simulink model "simple_double_argon_mask"  (Simulink 7.7)
settings: Solver=ode15s  StartTime=0.0  StopTime=3600*24  RelTol=1e-3
libraries: fl_lib x38, nesl_utility x5
settings Model: Creator=jlanfrey  LastModifiedBy=Administrateur

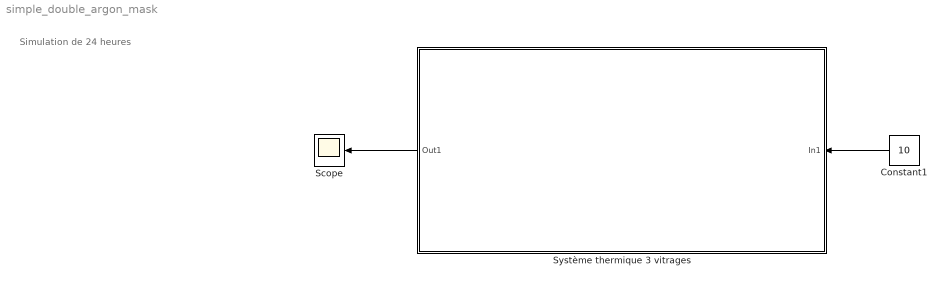
== system simple_double_argon_mask ==
  note: Simulation de 24 heures
  Constant1 : Constant  Value=10
  Scope : Scope
      settings: TimeRange=90000  YMin=14  YMax=20
  Système thermique 3 vitrages : Subsystem  mask{lf=0.6, hf=1, ev=4, ei=16, sp=10, hp=2.5, temp=20}
      mask prompts: lf "Largeur fenetre ? (m)"; hf "Hauteur fenetre ? (m)"; ev "Epaisseur d'un verre de la fenetre ? (mm)"; ei "Epaisseur isolant (air ou argon) ? (mm)"; sp "Suface pièce (m^2)"; hp "Hauteur pièce ? (m)"; temp "Température initiale (°C)"
      mask Display:
      | image(imread('vitrage.jpg'))
      | port_label('output', 1, 'Temp int')
      | port_label('input', 1, 'Temp exter')
  wires:
  Constant1/1 -> Système thermique 3 vitrages/1(In1)
  Système thermique 3 vitrages/1(Out1) -> Scope/1

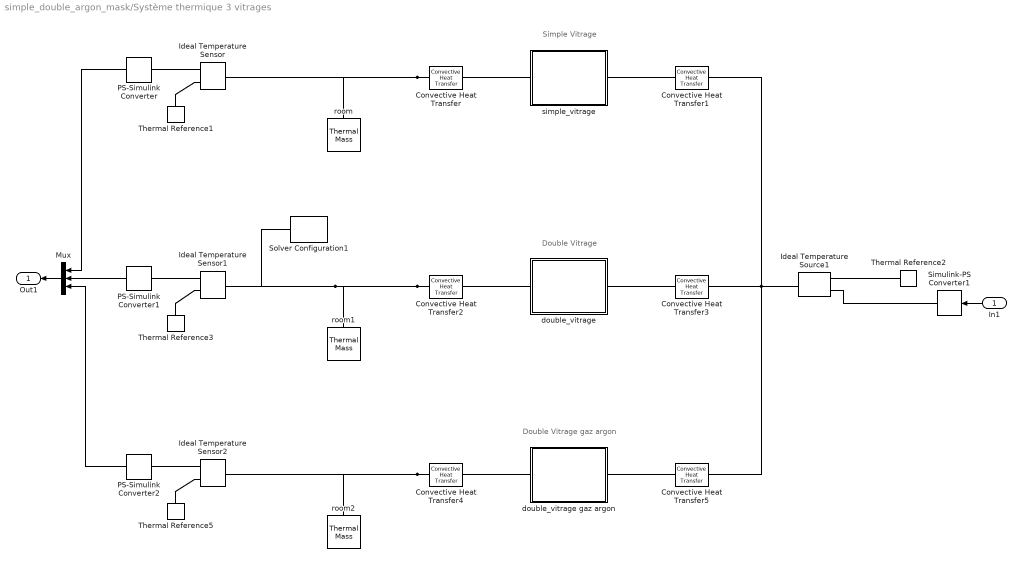
== system simple_double_argon_mask/Système thermique 3 vitrages ==
  note: Double Vitrage gaz argon
  note: Double Vitrage
  note: Simple Vitrage
  In1 : Inport
  Convective Heat Transfer : fl_lib/Thermal/Thermal Elements/Convective Heat Transfer  SystemSampleTime=-1  area=lf*hf m^2  heat_tr_coeff=1/0.13 W/(m^2 * K)  Q_Log=off  T_Log=off  LocalVarNames=|Q|T  LocalVarDescs=|Q|T  LocalVarLogging=[0 0]
  Convective Heat Transfer1 : fl_lib/Thermal/Thermal Elements/Convective Heat Transfer  SystemSampleTime=-1  area=lf*hf m^2  heat_tr_coeff=1/0.04 W/(m^2 * K)  Q_Log=off  T_Log=off  LocalVarNames=|Q|T  LocalVarDescs=|Q|T  LocalVarLogging=[0 0]
  Convective Heat Transfer2 : fl_lib/Thermal/Thermal Elements/Convective Heat Transfer  SystemSampleTime=-1  area=lf*hf m^2  heat_tr_coeff=1/0.13 W/(m^2 * K)  Q_Log=off  T_Log=off  LocalVarNames=|Q|T  LocalVarDescs=|Q|T  LocalVarLogging=[0 0]
  Convective Heat Transfer3 : fl_lib/Thermal/Thermal Elements/Convective Heat Transfer  SystemSampleTime=-1  area=lf*hf m^2  heat_tr_coeff=1/0.04 W/(m^2 * K)  Q_Log=off  T_Log=off  LocalVarNames=|Q|T  LocalVarDescs=|Q|T  LocalVarLogging=[0 0]
  Convective Heat Transfer4 : fl_lib/Thermal/Thermal Elements/Convective Heat Transfer  SystemSampleTime=-1  area=lf*hf m^2  heat_tr_coeff=1/0.13 W/(m^2 * K)  Q_Log=off  T_Log=off  LocalVarNames=|Q|T  LocalVarDescs=|Q|T  LocalVarLogging=[0 0]
  Convective Heat Transfer5 : fl_lib/Thermal/Thermal Elements/Convective Heat Transfer  SystemSampleTime=-1  area=lf*hf m^2  heat_tr_coeff=1/0.04 W/(m^2 * K)  Q_Log=off  T_Log=off  LocalVarNames=|Q|T  LocalVarDescs=|Q|T  LocalVarLogging=[0 0]
  Ideal Temperature Sensor : fl_lib/Thermal/Thermal Sensors/Ideal Temperature Sensor  SystemSampleTime=-1  Qs_Log=off  Ts_Log=off  LocalVarNames=|Qs|Ts  LocalVarDescs=|Qs|Ts  LocalVarLogging=[0 0]
  Ideal Temperature Sensor1 : fl_lib/Thermal/Thermal Sensors/Ideal Temperature Sensor  SystemSampleTime=-1  Qs_Log=off  Ts_Log=off  LocalVarNames=|Qs|Ts  LocalVarDescs=|Qs|Ts  LocalVarLogging=[0 0]
  Ideal Temperature Sensor2 : fl_lib/Thermal/Thermal Sensors/Ideal Temperature Sensor  SystemSampleTime=-1  Qs_Log=off  Ts_Log=off  LocalVarNames=|Qs|Ts  LocalVarDescs=|Qs|Ts  LocalVarLogging=[0 0]
  Ideal Temperature Source1 : fl_lib/Thermal/Thermal Sources/Ideal Temperature Source  SystemSampleTime=-1  Q_Log=off  T_Log=off  LocalVarNames=|Q|T  LocalVarDescs=|Q|T  LocalVarLogging=[0 0]
  Mux : Mux  Inputs=3
  PS-Simulink Converter : nesl_utility/PS-Simulink Converter  SystemSampleTime=-1  PhysicalDomain=network_engine_domain  LeftPortType=input  RightPortType=output  SubClassName=ps_output  Unit=C  AffineConversion=on
  PS-Simulink Converter1 : nesl_utility/PS-Simulink Converter  SystemSampleTime=-1  PhysicalDomain=network_engine_domain  LeftPortType=input  RightPortType=output  SubClassName=ps_output  Unit=C  AffineConversion=on
  PS-Simulink Converter2 : nesl_utility/PS-Simulink Converter  SystemSampleTime=-1  PhysicalDomain=network_engine_domain  LeftPortType=input  RightPortType=output  SubClassName=ps_output  Unit=C  AffineConversion=on
  Simulink-PS Converter1 : nesl_utility/Simulink-PS Converter  SystemSampleTime=-1  PhysicalDomain=network_engine_domain  LeftPortType=input  RightPortType=output  SubClassName=ps_input  Unit=C  AffineConversion=on  InputFilterTimeConstant=.001  UdotUserProvided=0
  Solver Configuration1 : nesl_utility/Solver Configuration  SystemSampleTime=-1  PhysicalDomain=network_engine_domain  LeftPortType=input  RightPortType=generic  SubClassName=solver  Accelerate=off  Profile=off  ResidualTolerance=1e-9  MaxNonlinIter=3  MaxModeIter=2  DoFixedCost=off  UseLocalSampling=off  DoDC=off  LinearAlgebra=Sparse  LocalSolverSampleTime=.001  LocalSolverChoice=NE_BACKWARD_EULER_ADVANCER  UseLocalSolver=off
  Thermal Reference{1..3,5} (4 alike) : fl_lib/Thermal/Thermal Elements/Thermal Reference  SystemSampleTime=-1  Q_Log=off  LocalVarNames=|Q  LocalVarDescs=|Q  LocalVarLogging=0
  double_vitrage : Subsystem
  double_vitrage gaz argon : Subsystem
  room : fl_lib/Thermal/Thermal Elements/Thermal Mass  SystemSampleTime=-1  mass=1.204*sp*hp kg  sp_heat=1004 J/kg/K  init_temp=temp C  Q_Log=off  LocalVarNames=|Q  LocalVarDescs=|Q  LocalVarLogging=0
  room1 : fl_lib/Thermal/Thermal Elements/Thermal Mass  SystemSampleTime=-1  mass=1.204*sp*hp kg  sp_heat=1004 J/kg/K  init_temp=temp C  Q_Log=off  LocalVarNames=|Q  LocalVarDescs=|Q  LocalVarLogging=0
  room2 : fl_lib/Thermal/Thermal Elements/Thermal Mass  SystemSampleTime=-1  mass=1.204*sp*hp kg  sp_heat=1004 J/kg/K  init_temp=temp C  Q_Log=off  LocalVarNames=|Q  LocalVarDescs=|Q  LocalVarLogging=0
  simple_vitrage : Subsystem
  Out1 : Outport
  wires:
  PS-Simulink Converter2/1 -> Mux/3
  PS-Simulink Converter1/1 -> Mux/2
  PS-Simulink Converter/1 -> Mux/1
  Mux/1 -> Out1/1
  In1/1 -> Simulink-PS Converter1/1
  connections:
  Convective Heat Transfer/LConn1 -- Ideal Temperature Sensor/LConn1 -- room/LConn1
  Convective Heat Transfer/RConn1 -- simple_vitrage/LConn1
  Convective Heat Transfer1/LConn1 -- simple_vitrage/RConn1
  Convective Heat Transfer5/RConn1 -- Convective Heat Transfer1/RConn1 -- Convective Heat Transfer3/RConn1 -- Ideal Temperature Source1/LConn1
  Convective Heat Transfer2/LConn1 -- room1/LConn1 -- Ideal Temperature Sensor1/LConn1 -- Solver Configuration1/RConn1
  Convective Heat Transfer2/RConn1 -- double_vitrage/LConn1
  Convective Heat Transfer3/LConn1 -- double_vitrage/RConn1
  Convective Heat Transfer4/LConn1 -- room2/LConn1 -- Ideal Temperature Sensor2/LConn1
  Convective Heat Transfer4/RConn1 -- double_vitrage gaz argon/LConn1
  Convective Heat Transfer5/LConn1 -- double_vitrage gaz argon/RConn1
  Thermal Reference1/LConn1 -- Ideal Temperature Sensor/RConn1
  PS-Simulink Converter/LConn1 -- Ideal Temperature Sensor/RConn2
  Thermal Reference3/LConn1 -- Ideal Temperature Sensor1/RConn1
  PS-Simulink Converter1/LConn1 -- Ideal Temperature Sensor1/RConn2
  Thermal Reference5/LConn1 -- Ideal Temperature Sensor2/RConn1
  PS-Simulink Converter2/LConn1 -- Ideal Temperature Sensor2/RConn2
  Simulink-PS Converter1/RConn1 -- Ideal Temperature Source1/RConn1
  Thermal Reference2/LConn1 -- Ideal Temperature Source1/RConn2

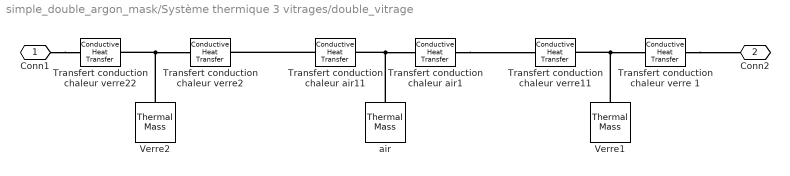
== system simple_double_argon_mask/Système thermique 3 vitrages/double_vitrage ==
  Transfert conduction chaleur air1 : fl_lib/Thermal/Thermal Elements/Conductive Heat Transfer  SystemSampleTime=-1  area=lf*hf m^2  thickness=ei/2 mm  th_cond=0.0262 W/(m*K)  Q_Log=off  T_Log=off  LocalVarNames=|Q|T  LocalVarDescs=|Q|T  LocalVarLogging=[0 0]
  Transfert conduction chaleur air11 : fl_lib/Thermal/Thermal Elements/Conductive Heat Transfer  SystemSampleTime=-1  area=lf*hf m^2  thickness=ei/2 mm  th_cond=0.0262 W/(m*K)  Q_Log=off  T_Log=off  LocalVarNames=|Q|T  LocalVarDescs=|Q|T  LocalVarLogging=[0 0]
  Transfert conduction chaleur verre 1 : fl_lib/Thermal/Thermal Elements/Conductive Heat Transfer  SystemSampleTime=-1  area=lf*hf m^2  thickness=ev/2 mm  th_cond=1.2 W/(m*K)  Q_Log=off  T_Log=off  LocalVarNames=|Q|T  LocalVarDescs=|Q|T  LocalVarLogging=[0 0]
  Transfert conduction chaleur verre11 : fl_lib/Thermal/Thermal Elements/Conductive Heat Transfer  SystemSampleTime=-1  area=lf*hf m^2  thickness=ev/2 mm  th_cond=1.2 W/(m*K)  Q_Log=off  T_Log=off  LocalVarNames=|Q|T  LocalVarDescs=|Q|T  LocalVarLogging=[0 0]
  Transfert conduction chaleur verre2 : fl_lib/Thermal/Thermal Elements/Conductive Heat Transfer  SystemSampleTime=-1  area=lf*hf m^2  thickness=ev/2 mm  th_cond=1.2 W/(m*K)  Q_Log=off  T_Log=off  LocalVarNames=|Q|T  LocalVarDescs=|Q|T  LocalVarLogging=[0 0]
  Transfert conduction chaleur verre22 : fl_lib/Thermal/Thermal Elements/Conductive Heat Transfer  SystemSampleTime=-1  area=lf*hf m^2  thickness=ev/2 mm  th_cond=1.2 W/(m*K)  Q_Log=off  T_Log=off  LocalVarNames=|Q|T  LocalVarDescs=|Q|T  LocalVarLogging=[0 0]
  Verre1 : fl_lib/Thermal/Thermal Elements/Thermal Mass  SystemSampleTime=-1  mass=lf*hf*ev*1e-3*2530 kg  sp_heat=720 J/kg/K  init_temp=temp C  Q_Log=off  LocalVarNames=|Q  LocalVarDescs=|Q  LocalVarLogging=0
  Verre2 : fl_lib/Thermal/Thermal Elements/Thermal Mass  SystemSampleTime=-1  mass=lf*hf*ev*1e-3*2530 kg  sp_heat=720 J/kg/K  init_temp=temp C  Q_Log=off  LocalVarNames=|Q  LocalVarDescs=|Q  LocalVarLogging=0
  air : fl_lib/Thermal/Thermal Elements/Thermal Mass  SystemSampleTime=-1  mass=lf*hf*ei*1e-3*1.204 kg  sp_heat=1004 J/kg/K  init_temp=temp C  Q_Log=off  LocalVarNames=|Q  LocalVarDescs=|Q  LocalVarLogging=0
  Conn1 : PMIOPort  Port=1  Side=Left
  Conn2 : PMIOPort  Port=2  Side=Right
  connections:
  Conn1/RConn1 -- Transfert conduction chaleur verre22/LConn1
  Verre2/LConn1 -- Transfert conduction chaleur verre22/RConn1 -- Transfert conduction chaleur verre2/LConn1
  Verre1/LConn1 -- Transfert conduction chaleur verre 1/LConn1 -- Transfert conduction chaleur verre11/RConn1
  Transfert conduction chaleur verre 1/RConn1 -- Conn2/RConn1
  Transfert conduction chaleur air11/LConn1 -- Transfert conduction chaleur verre2/RConn1
  Transfert conduction chaleur air1/RConn1 -- Transfert conduction chaleur verre11/LConn1
  air/LConn1 -- Transfert conduction chaleur air11/RConn1 -- Transfert conduction chaleur air1/LConn1

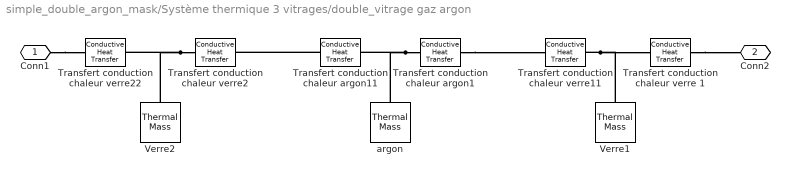
== system simple_double_argon_mask/Système thermique 3 vitrages/double_vitrage gaz argon ==
  Transfert conduction chaleur argon1 : fl_lib/Thermal/Thermal Elements/Conductive Heat Transfer  SystemSampleTime=-1  area=lf*hf m^2  thickness=ei/2 mm  th_cond=0.01772 W/(m*K)  Q_Log=off  T_Log=off  LocalVarNames=|Q|T  LocalVarDescs=|Q|T  LocalVarLogging=[0 0]
  Transfert conduction chaleur argon11 : fl_lib/Thermal/Thermal Elements/Conductive Heat Transfer  SystemSampleTime=-1  area=lf*hf m^2  thickness=ei/2 mm  th_cond=0.01772 W/(m*K)  Q_Log=off  T_Log=off  LocalVarNames=|Q|T  LocalVarDescs=|Q|T  LocalVarLogging=[0 0]
  Transfert conduction chaleur verre 1 : fl_lib/Thermal/Thermal Elements/Conductive Heat Transfer  SystemSampleTime=-1  area=lf*hf m^2  thickness=ev/2 mm  th_cond=1.2 W/(m*K)  Q_Log=off  T_Log=off  LocalVarNames=|Q|T  LocalVarDescs=|Q|T  LocalVarLogging=[0 0]
  Transfert conduction chaleur verre11 : fl_lib/Thermal/Thermal Elements/Conductive Heat Transfer  SystemSampleTime=-1  area=lf*hf m^2  thickness=ev/2 mm  th_cond=1.2 W/(m*K)  Q_Log=off  T_Log=off  LocalVarNames=|Q|T  LocalVarDescs=|Q|T  LocalVarLogging=[0 0]
  Transfert conduction chaleur verre2 : fl_lib/Thermal/Thermal Elements/Conductive Heat Transfer  SystemSampleTime=-1  area=lf*hf m^2  thickness=ev/2 mm  th_cond=1.2 W/(m*K)  Q_Log=off  T_Log=off  LocalVarNames=|Q|T  LocalVarDescs=|Q|T  LocalVarLogging=[0 0]
  Transfert conduction chaleur verre22 : fl_lib/Thermal/Thermal Elements/Conductive Heat Transfer  SystemSampleTime=-1  area=lf*hf m^2  thickness=ev/2 mm  th_cond=1.2 W/(m*K)  Q_Log=off  T_Log=off  LocalVarNames=|Q|T  LocalVarDescs=|Q|T  LocalVarLogging=[0 0]
  Verre1 : fl_lib/Thermal/Thermal Elements/Thermal Mass  SystemSampleTime=-1  mass=lf*hf*ev*1e-3*2530 kg  sp_heat=720 J/kg/K  init_temp=temp C  Q_Log=off  LocalVarNames=|Q  LocalVarDescs=|Q  LocalVarLogging=0
  Verre2 : fl_lib/Thermal/Thermal Elements/Thermal Mass  SystemSampleTime=-1  mass=lf*hf*ev*1e-3*2530 kg  sp_heat=720 J/kg/K  init_temp=temp C  Q_Log=off  LocalVarNames=|Q  LocalVarDescs=|Q  LocalVarLogging=0
  argon : fl_lib/Thermal/Thermal Elements/Thermal Mass  SystemSampleTime=-1  mass=lf*hf*ei*1e-3*1.783 kg  sp_heat=320 J/kg/K  init_temp=temp C  Q_Log=off  LocalVarNames=|Q  LocalVarDescs=|Q  LocalVarLogging=0
  Conn1 : PMIOPort  Port=1  Side=Left
  Conn2 : PMIOPort  Port=2  Side=Right
  connections:
  Conn1/RConn1 -- Transfert conduction chaleur verre22/LConn1
  Transfert conduction chaleur verre2/LConn1 -- Verre2/LConn1 -- Transfert conduction chaleur verre22/RConn1
  Transfert conduction chaleur verre11/RConn1 -- Verre1/LConn1 -- Transfert conduction chaleur verre 1/LConn1
  Transfert conduction chaleur argon1/LConn1 -- argon/LConn1 -- Transfert conduction chaleur argon11/RConn1
  Transfert conduction chaleur argon11/LConn1 -- Transfert conduction chaleur verre2/RConn1
  Transfert conduction chaleur argon1/RConn1 -- Transfert conduction chaleur verre11/LConn1
  Transfert conduction chaleur verre 1/RConn1 -- Conn2/RConn1

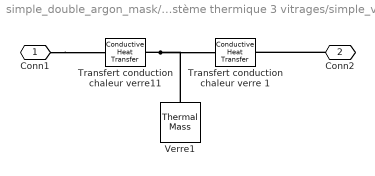
== system simple_double_argon_mask/Système thermique 3 vitrages/simple_vitrage ==
  Transfert conduction chaleur verre 1 : fl_lib/Thermal/Thermal Elements/Conductive Heat Transfer  SystemSampleTime=-1  area=lf*hf m^2  thickness=ev/2 mm  th_cond=1.2 W/(m*K)  Q_Log=off  T_Log=off  LocalVarNames=|Q|T  LocalVarDescs=|Q|T  LocalVarLogging=[0 0]
  Transfert conduction chaleur verre11 : fl_lib/Thermal/Thermal Elements/Conductive Heat Transfer  SystemSampleTime=-1  area=lf*hf m^2  thickness=ev/2 mm  th_cond=1.2 W/(m*K)  Q_Log=off  T_Log=off  LocalVarNames=|Q|T  LocalVarDescs=|Q|T  LocalVarLogging=[0 0]
  Verre1 : fl_lib/Thermal/Thermal Elements/Thermal Mass  SystemSampleTime=-1  mass=lf*hf*ev*1e-3*2530 kg  sp_heat=720 J/kg/K  init_temp=temp C  Q_Log=off  LocalVarNames=|Q  LocalVarDescs=|Q  LocalVarLogging=0
  Conn1 : PMIOPort  Port=1  Side=Left
  Conn2 : PMIOPort  Port=2  Side=Right
  connections:
  Conn1/RConn1 -- Transfert conduction chaleur verre11/LConn1
  Conn2/RConn1 -- Transfert conduction chaleur verre 1/RConn1
  Transfert conduction chaleur verre11/RConn1 -- Verre1/LConn1 -- Transfert conduction chaleur verre 1/LConn1
